simulink subsystem "PvtSubSys_VSM_ESS"  (R2020b)
settings: Solver=VariableStepAuto  StartTime=0.0  StopTime=10.0  RelTol=1e-3
values from neighbouring files (symbols this model uses):
  P_VSM_ESS_AccelPed_enable = 1.0    [ESS.sldd]
  P_VSM_ESS_AccPedlPosn_Param = 60.0    [ESS.sldd]
  P_VSM_ESS_ACtiveTime = 5.0    [ESS.sldd]
  P_VSM_ESS_AEBFlag_enable = 1.0    [ESS.sldd]
  P_VSM_ESS_AngleSpdTable_deg : value not decoded    [ESS.sldd]
  P_VSM_ESS_DangerPlausLeft = 0.3    [ESS.sldd]
  P_VSM_ESS_DangerPlausRight = 0.3    [ESS.sldd]
  P_VSM_ESS_DelayTime = 3.0    [ESS.sldd]
  P_VSM_ESS_DoorSts_enable = 1.0    [ESS.sldd]
  P_VSM_ESS_DriveIn : value not decoded    [ESS.sldd]
  P_VSM_ESS_DriveIn_BP : value not decoded    [ESS.sldd]
  P_VSM_ESS_DriverInputdSameDire_delaytime = 1.0    [ESS.sldd]
  P_VSM_ESS_DriverInputTrq_Param : value not decoded    [ESS.sldd]
  P_VSM_ESS_DrvOverTime_Param = 0.2    [ESS.sldd]
  P_VSM_ESS_DrvOverTime_Paramsame = 0.2    [ESS.sldd]
  P_VSM_ESS_DrvSBR_enable = 1.0    [ESS.sldd]
  P_VSM_ESS_ESPActive_enable = 1.0    [ESS.sldd]
  P_VSM_ESS_ESPFuncOffSts_enable = 1.0    [ESS.sldd]
  P_VSM_ESS_FcwDisFlag_enable = 1.0    [ESS.sldd]
  P_VSM_ESS_FcwSw_enable = 1.0    [ESS.sldd]
  P_VSM_ESS_HiLoBeam_enable = 1.0    [ESS.sldd]
  P_VSM_ESS_IPSpeed_kmh : value not decoded    [ESS.sldd]
  P_VSM_ESS_LateralAccel_enable = 1.0    [ESS.sldd]
  P_VSM_ESS_LgtAccelLower_Param = -8.0    [ESS.sldd]
  P_VSM_ESS_LgtAccelUpper_Param = 3.0    [ESS.sldd]
  P_VSM_ESS_MasterCylindBrake = 5.0    [ESS.sldd]
  P_VSM_ESS_MaxLateral_mss : value not decoded    [ESS.sldd]
  P_VSM_ESS_OVERRIDE_SW = 0.0    [ESS.sldd]
  P_VSM_ESS_SafeDistance_m = 1.5    [ESS.sldd]
  P_VSM_ESS_SpdPoint_kmh : value not decoded    [ESS.sldd]
  P_VSM_ESS_SpdTime_s : value not decoded    [ESS.sldd]
  P_VSM_ESS_SteerWheelSpd_BP : value not decoded    [ESS.sldd]
  P_VSM_ESS_SteerWheelSpd_enable = 1.0    [ESS.sldd]
  P_VSM_ESS_SteerWheelSpd_Param : value not decoded    [ESS.sldd]
  P_VSM_ESS_StopA0_Param = 0.2    [ESS.sldd]
  P_VSM_ESS_StopA1_Param = 0.02    [ESS.sldd]
  P_VSM_ESS_StopA1Time_Param = 2.0    [ESS.sldd]
  P_VSM_ESS_TrailerSts_enable = 1.0    [ESS.sldd]
  P_VSM_ESS_VehLgtAccel_enable = 1.0    [ESS.sldd]
  P_VSM_ESS_Vehspeed_enable = 1.0    [ESS.sldd]
  P_VSM_ESS_WiprReq_enable = 1.0    [ESS.sldd]
undefined symbols (not defined in the file or in its folder): P_Global_WheelBase_m
libraries: simulink x104, TrueDurationTime x6
(part 1 of 3)
settings Model: Creator=GW00133806  LastModifiedBy=GW00164938

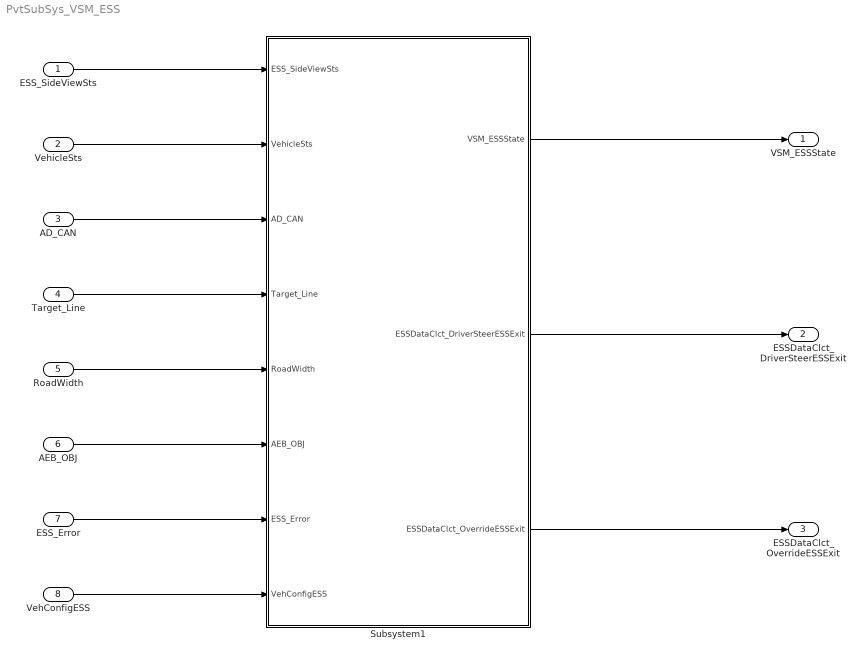
== system PvtSubSys_VSM_ESS ==
  ESS_SideViewSts : Inport  OutDataTypeStr=Bus: PLAN_DPC_ESS_BUS
  VehicleSts : Inport  Port=2  OutDataTypeStr=Bus: ESS_VehicleSts_BUS
  AD_CAN : Inport  Port=3
  Target_Line : Inport  Port=4  OutDataTypeStr=Bus: LSM_ESS_BUS
  RoadWidth : Inport  Port=5
  AEB_OBJ : Inport  Port=6  OutDataTypeStr=Bus: TOS_AEB_LONOBJ_BUS
  ESS_Error : Inport  Port=7
  VehConfigESS : Inport  Port=8
  Subsystem1 : Subsystem
  VSM_ESSState : Outport
  ESSDataClct_DriverSteerESSExit : Outport  Port=2
  ESSDataClct_OverrideESSExit : Outport  Port=3
  wires:
  RoadWidth/1 -> Subsystem1/5(RoadWidth)
  VehConfigESS/1 -> Subsystem1/8(VehConfigESS)
  ESS_Error/1 -> Subsystem1/7(ESS_Error)
  Subsystem1/2(ESSDataClct_DriverSteerESSExit) -> ESSDataClct_DriverSteerESSExit/1
  VehicleSts/1 -> Subsystem1/2(VehicleSts)
  Subsystem1/3(ESSDataClct_OverrideESSExit) -> ESSDataClct_OverrideESSExit/1
  ESS_SideViewSts/1 -> Subsystem1/1(ESS_SideViewSts)
  AEB_OBJ/1 -> Subsystem1/6(AEB_OBJ)
  Target_Line/1 -> Subsystem1/4(Target_Line)
  Subsystem1/1(VSM_ESSState) -> VSM_ESSState/1
  AD_CAN/1 -> Subsystem1/3(AD_CAN)

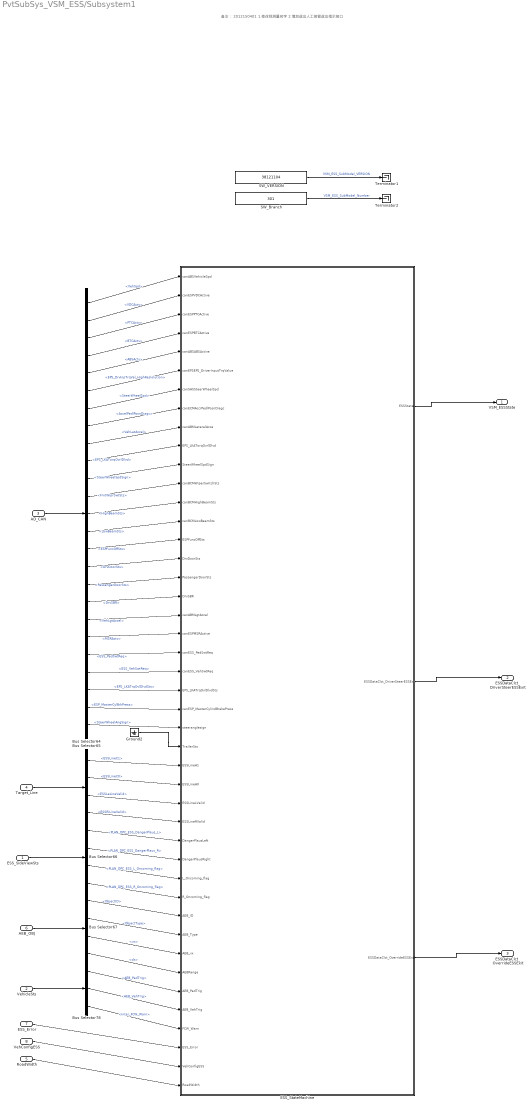
== system PvtSubSys_VSM_ESS/Subsystem1 ==
  note: 备注：
      | 2012150401
      |       1.修改观测量名字
      |       2.增加退出人工接管退出指示接口
  ESS_SideViewSts : Inport
  VehicleSts : Inport  Port=2
  AD_CAN : Inport  Port=3
  Target_Line : Inport  Port=4
  RoadWidth : Inport  Port=5
  AEB_OBJ : Inport  Port=6
  ESS_Error : Inport  Port=7
  VehConfigESS : Inport  Port=8
  Bus Selector64 : BusSelector  OutputSignals=VehSpd,VDCActv,PTCActv,BTCActv,ABSActv,EPS_DrvInpTrqVal_HighReslolution,SteerWheelSpd,AccelPedlPosnDiagc,VehLatAccel,EPS_LKATorqOvrlDlvd,SteerWheelSpdSign,FrntWiprSwtSts,HighBeamSts,LowBeamSts,ESPFuncOffSts,DrvDoorSts,PassengerDoorSts,DrvSBR,VehLgtAccel,MSRActv,ESS_PedSwtReq,ESS_VehSwtReq,EPS_LKATrqOvlDlvdSts,ESP_MasterCylBrkPress,SteerWheelAngSign
  Bus Selector65 : BusSelector  OutputSignals=ESSLineC1,ESSLineC0,ESSLeLineValid,ESSRiLineValid
  Bus Selector66 : BusSelector  OutputSignals=PLAN_DPC_ESS_DangerPlaus_L,PLAN_DPC_ESS_DangerPlaus_R,PLAN_DPC_ESS_L_Oncoming_flag,PLAN_DPC_ESS_R_Oncoming_flag
  Bus Selector67 : BusSelector  OutputSignals=ObjectID,ObjectType,vx,dx
  Bus Selector78 : BusSelector  OutputSignals=AEB_PedTrig,AEB_VehTrig,Inter_FCW_Warn
  ESS_StateMachine : Subsystem
  Ground2 : Ground
  SW_Branch : Constant  Value=301  OutDataTypeStr=uint16
  SW_VERSION : Constant  Value=38121104  OutDataTypeStr=uint32
  Terminator1 : Terminator
  Terminator2 : Terminator
  VSM_ESSState : Outport
  ESSDataClct_DriverSteerESSExit : Outport  Port=2
  ESSDataClct_OverrideESSExit : Outport  Port=3
  wires:
  SW_Branch/1 -> Terminator2/1  "VSM_ESS_SubModel_Number"
  Bus Selector65/3 -> ESS_StateMachine/29(ESSLineLValid)  "<ESSLeLineValid>"
  ESS_StateMachine/1(ESSState) -> VSM_ESSState/1
  Bus Selector64/3 -> ESS_StateMachine/3(canESPPTCActive)  "<PTCActv>"
  Bus Selector64/5 -> ESS_StateMachine/5(canABSABSActive)  "<ABSActv>"
  AD_CAN/1 -> Bus Selector64/1
  Bus Selector64/9 -> ESS_StateMachine/9(canABMLateralAcce)  "<VehLatAccel>"
  Bus Selector64/11 -> ESS_StateMachine/11(SteerWheelSpdSign)  "<SteerWheelSpdSign>"
  Bus Selector65/2 -> ESS_StateMachine/28(ESSLineA0)  "<ESSLineC0>"
  Bus Selector64/18 -> ESS_StateMachine/18(DrvSBR)  "<DrvSBR>"
  Bus Selector78/2 -> ESS_StateMachine/40(AEB_VehTrig)  "<AEB_VehTrig>"
  Bus Selector78/1 -> ESS_StateMachine/39(AEB_PedTrig)  "<AEB_PedTrig>"
  Bus Selector64/15 -> ESS_StateMachine/15(ESPFuncOffSts)  "<ESPFuncOffSts>"
  Bus Selector78/3 -> ESS_StateMachine/41(FCW_Warn)  "<Inter_FCW_Warn>"
  Bus Selector64/8 -> ESS_StateMachine/8(canECMAccrPedlPosnDiagc)  "<AccelPedlPosnDiagc>"
  Bus Selector64/20 -> ESS_StateMachine/20(canESPMSRActive)  "<MSRActv>"
  Bus Selector64/14 -> ESS_StateMachine/14(canBCMLowBeamSts)  "<LowBeamSts>"
  Bus Selector66/3 -> ESS_StateMachine/33(L_Oncoming_flag)  "<PLAN_DPC_ESS_L_Oncoming_flag>"
  Bus Selector67/4 -> ESS_StateMachine/38(AEBRange)  "<dx>"
  Target_Line/1 -> Bus Selector65/1
  ESS_SideViewSts/1 -> Bus Selector66/1
  Bus Selector64/2 -> ESS_StateMachine/2(canESPVDCActive)  "<VDCActv>"
  Bus Selector64/13 -> ESS_StateMachine/13(canBCMHighBeamSts)  "<HighBeamSts>"
  Bus Selector66/2 -> ESS_StateMachine/32(DangerPlausRight)  "<PLAN_DPC_ESS_DangerPlaus_R>"
  Bus Selector66/1 -> ESS_StateMachine/31(DangerPlausLeft)  "<PLAN_DPC_ESS_DangerPlaus_L>"
  Ground2/1 -> ESS_StateMachine/26(TrailerSts)
  Bus Selector64/7 -> ESS_StateMachine/7(canSASSteerWheelSpd)  "<SteerWheelSpd>"
  Bus Selector64/21 -> ESS_StateMachine/21(canESS_PedSwtReq)  "<ESS_PedSwtReq>"
  Bus Selector64/6 -> ESS_StateMachine/6(canEPSEPS_DriverInputTrqValue)  "<EPS_DrvInpTrqVal_HighReslolution>"
  Bus Selector67/1 -> ESS_StateMachine/35(AEB_ID)  "<ObjectID>"
  Bus Selector65/4 -> ESS_StateMachine/30(ESSLineRValid)  "<ESSRiLineValid>"
  Bus Selector67/2 -> ESS_StateMachine/36(AEB_Type)  "<ObjectType>"
  Bus Selector67/3 -> ESS_StateMachine/37(AEB_vx)  "<vx>"
  Bus Selector66/4 -> ESS_StateMachine/34(R_Oncoming_flag)  "<PLAN_DPC_ESS_R_Oncoming_flag>"
  Bus Selector64/12 -> ESS_StateMachine/12(canBCMWiperSwitchSts)  "<FrntWiprSwtSts>"
  Bus Selector64/16 -> ESS_StateMachine/16(DrvDoorSts)  "<DrvDoorSts>"
  Bus Selector64/1 -> ESS_StateMachine/1(canABSVehicleSpd)  "<VehSpd>"
  Bus Selector64/22 -> ESS_StateMachine/22(canESS_VehSwtReq)  "<ESS_VehSwtReq>"
  Bus Selector64/19 -> ESS_StateMachine/19(canABMLgtAccel)  "<VehLgtAccel>"
  Bus Selector65/1 -> ESS_StateMachine/27(ESSLineA1)  "<ESSLineC1>"
  Bus Selector64/17 -> ESS_StateMachine/17(PassengerDoorSts)  "<PassengerDoorSts>"
  AEB_OBJ/1 -> Bus Selector67/1
  Bus Selector64/4 -> ESS_StateMachine/4(canESPBTCActive)  "<BTCActv>"
  ESS_StateMachine/3(ESSDataClct_OverrideESSExit) -> ESSDataClct_OverrideESSExit/1
  ESS_StateMachine/2(ESSDataClct_DriverSteerESSExit) -> ESSDataClct_DriverSteerESSExit/1
  VehicleSts/1 -> Bus Selector78/1
  Bus Selector64/10 -> ESS_StateMachine/10(EPS_LKATorqOvrlDlvd)  "<EPS_LKATorqOvrlDlvd>"
  SW_VERSION/1 -> Terminator1/1  "VSM_ESS_SubModel_VERSION"
  ESS_Error/1 -> ESS_StateMachine/42(ESS_Error)
  VehConfigESS/1 -> ESS_StateMachine/43(VehConfigESS)
  RoadWidth/1 -> ESS_StateMachine/44(RoadWidth)
  Bus Selector64/23 -> ESS_StateMachine/23(EPS_LKATrqOvlDlvdSts)  "<EPS_LKATrqOvlDlvdSts>"
  Bus Selector64/24 -> ESS_StateMachine/24(canESP_MasterCylindBrakePress)  "<ESP_MasterCylBrkPress>"
  Bus Selector64/25 -> ESS_StateMachine/25(steeranglesign)  "<SteerWheelAngSign>"

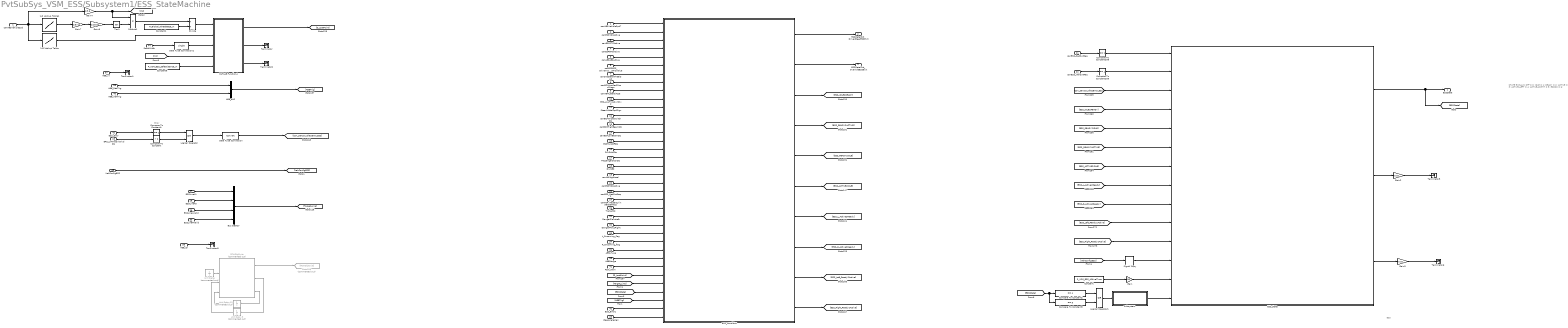
== system PvtSubSys_VSM_ESS/Subsystem1/ESS_StateMachine ==
  note: ESS
  note: STATE EXPLAIN:
      | OFF = 0;
      | IDLE = 1;
      | READY = 2;
      | ACTIVE = 3;
      | ACTIVE_LEFT = 4;
      | ACTIVE_RIGHT = 5;
      | ERROR = 6;
  note: Error
  canABSVehicleSpd : Inport
  canESPVDCActive : Inport  Port=2
  canESPPTCActive : Inport  Port=3
  canESPBTCActive : Inport  Port=4
  canABSABSActive : Inport  Port=5
  canEPSEPS_DriverInputTrqValue : Inport  Port=6
  canSASSteerWheelSpd : Inport  Port=7
  canECMAccrPedlPosnDiagc : Inport  Port=8
  canABMLateralAcce : Inport  Port=9
  EPS_LKATorqOvrlDlvd : Inport  Port=10
  SteerWheelSpdSign : Inport  Port=11
  canBCMWiperSwitchSts : Inport  Port=12
  canBCMHighBeamSts : Inport  Port=13
  canBCMLowBeamSts : Inport  Port=14
  ESPFuncOffSts : Inport  Port=15
  DrvDoorSts : Inport  Port=16
  PassengerDoorSts : Inport  Port=17
  DrvSBR : Inport  Port=18
  canABMLgtAccel : Inport  Port=19
  canESPMSRActive : Inport  Port=20
  canESS_PedSwtReq : Inport  Port=21
  canESS_VehSwtReq : Inport  Port=22
  EPS_LKATrqOvlDlvdSts : Inport  Port=23
  canESP_MasterCylindBrakePress : Inport  Port=24
  steeranglesign : Inport  Port=25
  TrailerSts : Inport  Port=26
  ESSLineA1 : Inport  Port=27
  ESSLineA0 : Inport  Port=28
  ESSLineLValid : Inport  Port=29
  ESSLineRValid : Inport  Port=30
  DangerPlausLeft : Inport  Port=31
  DangerPlausRight : Inport  Port=32
  L_Oncoming_flag : Inport  Port=33
  R_Oncoming_flag : Inport  Port=34
  AEB_ID : Inport  Port=35
  AEB_Type : Inport  Port=36
  AEB_vx : Inport  Port=37
  AEBRange : Inport  Port=38
  AEB_PedTrig : Inport  Port=39
  AEB_VehTrig : Inport  Port=40
  FCW_Warn : Inport  Port=41
  ESS_Error : Inport  Port=42
  VehConfigESS : Inport  Port=43
  RoadWidth : Inport  Port=44
  1-D Lookup Table : Lookup_n-D  NumberOfTableDimensions=1  BreakpointsForDimension1=P_VSM_ESS_SpdPoint_kmh  Table=P_VSM_ESS_SpdTime_s  InternalRulePriority=Speed  RndMeth=Simplest  InputSameDT=on
  1-D Lookup Table1 : Lookup_n-D  NumberOfTableDimensions=1  BreakpointsForDimension1=P_VSM_ESS_SpdPoint_kmh  Table=P_VSM_ESS_AngleSpdTable_deg  InternalRulePriority=Speed  RndMeth=Simplest  InputSameDT=on
  AEB_BUS : BusCreator  Inputs=2
  Bus Creator : BusCreator  Inputs=4
  Compare To Constant : simulink/Logic and Bit Operations/Compare To Constant  relop=>  const=2  OutDataTypeStr=boolean
  Compare To Constant1 : simulink/Logic and Bit Operations/Compare To Constant  relop===  const=1  OutDataTypeStr=boolean
  Compare To Constant2 : simulink/Logic and Bit Operations/Compare To Constant  relop===  const=4  OutDataTypeStr=boolean
  Compare To Constant208 : simulink/Logic and Bit Operations/Compare To Constant  relop===  const=1  OutDataTypeStr=boolean
  Compare To Constant209 : simulink/Logic and Bit Operations/Compare To Constant  relop===  const=1  OutDataTypeStr=boolean
  Compare To Constant3 : simulink/Logic and Bit Operations/Compare To Constant  relop===  const=5  OutDataTypeStr=boolean
  Constant : Constant  Value=P_VSM_ESS_ACtiveTime
  Constant1 : Constant  Value=P_Global_WheelBase_m
  Constant6 : Constant  Value=P_VSM_ESS_SafeDistance_m
  Data Type Conversion : DataTypeConversion
  Data Type Conversion2 : DataTypeConversion  OutDataTypeStr=single
  Divide : Product  Inputs=*/
  ESS_Condition : Subsystem
  ESS_Error1 : InportShadow  Port=42
  ESS_State : Stateflow chart  TreatAsAtomicUnit=on
  FCWObjExist : MATLAB Function  Commented=on  TreatAsAtomicUnit=on
  Gain : Gain  Gain=50
  Gain2 : Gain  Gain=0.02  OutDataTypeStr=single
  Gain3 : Gain  Gain=0.02  OutDataTypeStr=single
  Gain4 : Gain  Gain=1/3.6
  Gain7 : Gain  Gain=1/57.3
  Gain8 : Gain  Gain=1/18.02
  Goto158 : Goto  Commented=on  GotoTag=FCWObjExist
  Logical Operator : Logic  Operator=OR  AllPortsSameDT=off  OutDataTypeStr=boolean
  Logical Operator1 : Logic  Operator=OR  AllPortsSameDT=off  OutDataTypeStr=boolean
  MATLAB Function4 : MATLAB Function  TreatAsAtomicUnit=on
  Product1 : Product
  Signal Copy : SignalConversion  OverrideOpt=off
  Subsystem : Subsystem
  Tan1 : Trigonometry  Operator=tan
  Terminator{,1..3,5..6} (6 alike) : Terminator
  Unit Delay : UnitDelay  Commented=on  SampleTime=-1  HasFrameUpgradeWarning=on
  Unit Delay13 : UnitDelay  Commented=on  SampleTime=-1  HasFrameUpgradeWarning=on
  Unit Delay3 : UnitDelay  Commented=on  SampleTime=-1  HasFrameUpgradeWarning=on
  canABSVehicleSpd7 : InportShadow
  canESS_PedSwtReq2 : InportShadow  Port=21
  ESSState : Outport
  ESSDataClct_DriverSteerESSExit : Outport  Port=2
  ESSDataClct_OverrideESSExit : Outport  Port=3
  wires:
  Subsystem/1(DelayReady) -> ESS_State/14(delaytime)  "VSM_ESS_DelayReady"
  Compare To Constant3/1 -> Logical Operator1/2
  Compare To Constant2/1 -> Logical Operator1/1
  [ESSState] -> Compare To Constant2/1, Compare To Constant3/1
  Logical Operator1/1 -> Subsystem/1(ESSAct)
  ESS_State/3(L) -> Gain3/1
  Gain3/1 -> Terminator6/1  "VSM_ESS_StateL"
  Gain2/1 -> Terminator5/1  "VSM_ESS_StateR"
  ESS_State/2(R) -> Gain2/1
  ESS_Error1/1 -> ESS_Condition/35(Dia_inhibit)
  Compare To Constant1/1 -> Logical Operator/1
  [VehConfigESS] -> Signal Copy/1
  [ESS_READY2IDLE] -> ESS_State/5(ESS_READY2IDLE)  "VSM_ESS_READY2IDLE"
  Compare To Constant209/1 -> ESS_State/2(ESS_VehSwtReq)  "VSM_ESS_VehSwtReq"
  [ESS_Right_Ready2Active] -> ESS_State/11(ESS_RIGHT_READY2ACTIVE)  "VSM_ESS_Right_READY2ACTIVE"
  [ESS_READY2ACTIVE] -> ESS_State/6(ESS_READY2ACTIVE)  "VSM_ESS_READY2ACTIVE"
  [Con_Sensor_Idle2Error_ESS] -> ESS_State/3(ERROR)  "VSM_ESS_Sensor_idle2error"
  canESS_VehSwtReq/1 -> Compare To Constant209/1
  [ESS_ACTIVE2IDLE] -> ESS_State/7(ESS_ACTIVE2IDLE)  "VSM_ESS_ACTIVE2IDLE"
  canESS_PedSwtReq/1 -> Compare To Constant208/1
  [ESS_L_Active2Ready] -> ESS_State/8(ESS_L_ACTIVE2READY)  "VSM_ESS_L_ACTIVE2READY"
  [ESS_R_Active2Ready] -> ESS_State/9(ESS_R_ACTIVE2READY)  "VSM_ESS_R_ACTIVE2READY"
  [ESS_IDLE2READY] -> ESS_State/4(ESS_IDLE2READY)  "VSM_ESS_IDLE2READY"
  Compare To Constant208/1 -> ESS_State/1(ESS_PedSwtReq)  "VSM_ESS_PedSwtReq"
  [ESS_Left_Ready2Active] -> ESS_State/10(ESS_LEFT_READY2ACTIVE)  "VSM_ESS_Left_READY2ACTIVE"
  MATLAB Function4/1(Dmin) -> [D_LastPoint]  "VSM_ESS_LastPoint"
  AEB_BUS/1 -> [AEBTrig]
  AEB_PedTrig/1 -> AEB_BUS/1
  AEB_vx/1 -> Terminator1/1
  AEB_VehTrig/1 -> AEB_BUS/2
  FCWObjExist/3(counter) -> Unit Delay13/1
  Unit Delay/1 -> FCWObjExist/2(pre_FCWObjID)
  Unit Delay3/1 -> FCWObjExist/3(pre_ESS_act_ID)
  Unit Delay13/1 -> FCWObjExist/4(pre_counter)
  FCWObjExist/2(ESS_act_ID) -> Unit Delay3/1
  ESSLineA1/1 -> Bus Creator/1  "ESSLineA1"
  ESSLineA0/1 -> Bus Creator/2  "ESSLineA0"
  ESSLineLValid/1 -> Bus Creator/3  "ESSLineLValid"
  ESSLineRValid/1 -> Bus Creator/4  "ESSLineRValid"
  Bus Creator/1 -> [Target_Line]
  FCWObjExist/1(FCWObjExist) -> Goto158/1
  ? -> FCWObjExist/1(FCWObjID), Unit Delay/1
  ESS_State/1(ESS_STATE) -> ESSState/1, [ESSState]  "VSM_ESSState"
  canABSVehicleSpd7/1 -> ESS_Condition/1(canABSVehicleSpd)
  canESPVDCActive/1 -> ESS_Condition/2(canESPVDCActive)
  canESPPTCActive/1 -> ESS_Condition/3(canESPPTCActive)
  canESPBTCActive/1 -> ESS_Condition/4(canESPBTCActive)
  canABSABSActive/1 -> ESS_Condition/5(canABSABSActive)
  canEPSEPS_DriverInputTrqValue/1 -> ESS_Condition/6(canEPSEPS_DriverInputTrqValue)
  canSASSteerWheelSpd/1 -> ESS_Condition/7(canSASSteerWheelSpd)
  canECMAccrPedlPosnDiagc/1 -> ESS_Condition/8(canECMAccrPedlPosnDiagc)
  canABMLateralAcce/1 -> ESS_Condition/9(canABMLateralAcce)
  EPS_LKATorqOvrlDlvd/1 -> ESS_Condition/10(Torq)
  SteerWheelSpdSign/1 -> ESS_Condition/11(SteerWheelSpdSign)
  canBCMWiperSwitchSts/1 -> ESS_Condition/12(canBCMWiperSwitchSts)
  canBCMHighBeamSts/1 -> ESS_Condition/13(canBCMHighBeamSts)
  canBCMLowBeamSts/1 -> ESS_Condition/14(canBCMLowBeamSts)
  ESPFuncOffSts/1 -> ESS_Condition/15(ESPFuncOffSts)
  DrvDoorSts/1 -> ESS_Condition/16(DrvDoorSts)
  PassengerDoorSts/1 -> ESS_Condition/17(PassengerDoorSts)
  DrvSBR/1 -> ESS_Condition/18(DrvSBR)
  canABMLgtAccel/1 -> ESS_Condition/19(canABMLgtAccel)
  canESPMSRActive/1 -> ESS_Condition/20(canESPMSRActive)
  canESS_PedSwtReq2/1 -> ESS_Condition/21(canESS_PedSwtReq)
  TrailerSts/1 -> ESS_Condition/23(TrailerSts)
  DangerPlausLeft/1 -> ESS_Condition/24(DangerPlausLeft)
  DangerPlausRight/1 -> ESS_Condition/25(DangerPlausRight)
  L_Oncoming_flag/1 -> ESS_Condition/26(L_Oncoming_flag)
  R_Oncoming_flag/1 -> ESS_Condition/27(R_Oncoming_flag)
  AEB_Type/1 -> ESS_Condition/28(AEB_Type)
  AEBRange/1 -> ESS_Condition/29(AEBRange)
  FCW_Warn/1 -> ESS_Condition/30(FCW_Warn)
  ESS_Condition/1(ESSDataClct_DriverSteerESSExit) -> ESSDataClct_DriverSteerESSExit/1
  ESS_Condition/2(ESSDataClct_OverrideESSExit) -> ESSDataClct_OverrideESSExit/1
  ESS_Condition/3(ESS_IDLE2READY) -> [ESS_IDLE2READY]
  ESS_Condition/4(ESS_READY2ACTIVE) -> [ESS_READY2ACTIVE]
  ESS_Condition/5(ESS_READY2IDLE) -> [ESS_READY2IDLE]
  ESS_Condition/6(ESS_ACTIVE2IDLE) -> [ESS_ACTIVE2IDLE]
  ESS_Condition/7(ESS_L_Active2Ready) -> [ESS_L_Active2Ready]
  ESS_Condition/8(ESS_R_Active2Ready) -> [ESS_R_Active2Ready]
  ESS_Condition/9(ESS_Left_Ready2Active) -> [ESS_Left_Ready2Active]
  ESS_Condition/10(ESS_Right_Ready2Active) -> [ESS_Right_Ready2Active]
  [D_LastPoint] -> ESS_Condition/31(D_LastPoint)
  [Target_Line] -> ESS_Condition/32(Target_Line)
  [AEBTrig] -> ESS_Condition/34(AEBTrig)
  [ESSState] -> ESS_Condition/33(ESSState)
  Signal Copy/1 -> ESS_State/12(VehConfigESS)  "VSM_ESS_VehCnfgESS"
  ESS_Error/1 -> Compare To Constant1/1
  VehConfigESS/1 -> [VehConfigESS]
  Data Type Conversion/1 -> [Con_Sensor_Idle2Error_ESS]
  MATLAB Function4/2(Tx) -> Terminator/1
  1-D Lookup Table1/1 -> Gain7/1
  Gain7/1 -> Gain8/1
  Gain8/1 -> Tan1/1
  Tan1/1 -> Product1/2
  Product1/1 -> Divide/1
  Divide/1 -> MATLAB Function4/1(angle)
  Gain4/1 -> [ms], Product1/1
  [ms] -> MATLAB Function4/4(V)
  1-D Lookup Table/1 -> MATLAB Function4/2(t)
  Constant6/1 -> MATLAB Function4/5(d)
  Logical Operator/1 -> Data Type Conversion/1
  EPS_LKATrqOvlDlvdSts/1 -> Compare To Constant/1
  Compare To Constant/1 -> Logical Operator/2
  RoadWidth/1 -> Data Type Conversion2/1
  canABSVehicleSpd/1 -> 1-D Lookup Table/1, Gain4/1, 1-D Lookup Table1/1
  Data Type Conversion2/1 -> MATLAB Function4/3(L)
  MATLAB Function4/3(D) -> Terminator2/1
  Constant1/1 -> Divide/2
  Constant/1 -> Gain/1
  Gain/1 -> ESS_State/13(ESS_ACtime)
  AEB_ID/1 -> Terminator3/1
  canESP_MasterCylindBrakePress/1 -> ESS_Condition/22(canESP_MasterCylindBrakePress)
  steeranglesign/1 -> ESS_Condition/36(steeranglesign)
